simulink model "Compensator"  (Simulink 6.1)
settings: Solver=ode45  StartTime=0.0  StopTime=10.0  RelTol=1e-3
libraries: dspmtrx3 x2
settings Model: LastModifiedBy=fhuang
settings DebuggingCC: SolverPrmCheckMsg=warning

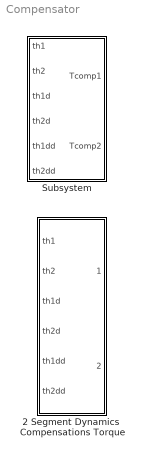
== system Compensator ==
  2 Segment Dynamics  Compensations Torque : Subsystem
  Subsystem : Subsystem

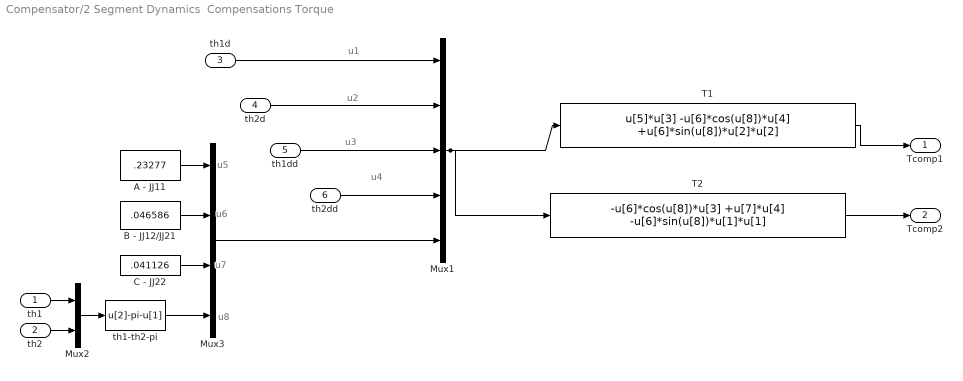
== system Compensator/2 Segment Dynamics  Compensations Torque ==
  note: u1
  note: u2
  note: u3
  note: u4
  note: u5
  note: u6
  note: u7
  note: u8
  th1 : Inport  Port=1  LatchInput=off
  th2 : Inport  Port=2  LatchInput=off
  th1d : Inport  Port=3  LatchInput=off
  th2d : Inport  Port=4  LatchInput=off
  th1dd : Inport  Port=5  LatchInput=off
  th2dd : Inport  Port=6  LatchInput=off
  A - JJ11 : Constant  Value=.23277
  B - JJ12/JJ21 : Constant  Value=.046586
  C - JJ22 : Constant  Value=.041126
  Mux1 : Mux  Inputs=5
  Mux2 : Mux  Inputs=2
  Mux3 : Mux
  T1 : Fcn  Expr="u[5]*u[3]   -u[6]*cos(u[8])*u[4]   +u[6]*sin(u[8])*u[2]*u[2]"
  T2 : Fcn  Expr="-u[6]*cos(u[8])*u[3]    +u[7]*u[4]    -u[6]*sin(u[8])*u[1]*u[1]"
  th1-th2-pi : Fcn  Expr=u[2]-pi-u[1]
  Tcomp1 : Outport
  Tcomp2 : Outport  Port=2
  wires:
  T1/1 -> Tcomp1/1
  Mux1/1 -> T1/1, T2/1
  Mux3/1 -> Mux1/5
  A - JJ11/1 -> Mux3/1
  B - JJ12/JJ21/1 -> Mux3/2
  C - JJ22/1 -> Mux3/3
  th1-th2-pi/1 -> Mux3/4
  th1d/1 -> Mux1/1
  th2d/1 -> Mux1/2
  th1dd/1 -> Mux1/3
  th2dd/1 -> Mux1/4
  th2/1 -> Mux2/2
  th1/1 -> Mux2/1
  Mux2/1 -> th1-th2-pi/1
  T2/1 -> Tcomp2/1

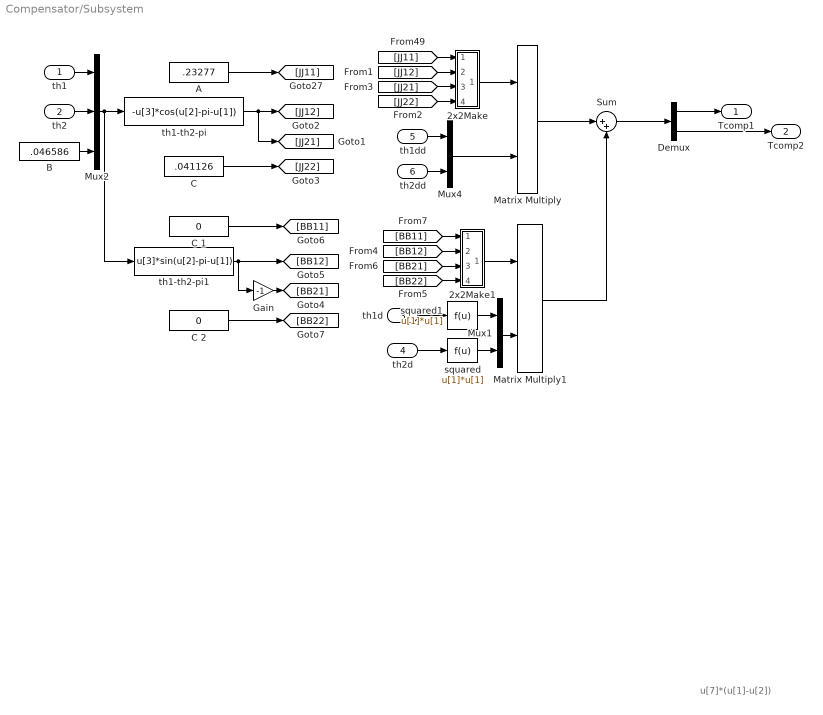
== system Compensator/Subsystem ==
  note: u[7]*(u[1]-u[2])
  th1 : Inport  Port=1  LatchInput=off
  th2 : Inport  Port=2  LatchInput=off
  th1d : Inport  Port=3  LatchInput=off
  th2d : Inport  Port=4  LatchInput=off
  th1dd : Inport  Port=5  LatchInput=off
  th2dd : Inport  Port=6  LatchInput=off
  2x2Make : Subsystem
  2x2Make1 : Subsystem
  A : Constant  Value=.23277
  B : Constant  Value=.046586
  "C " : Constant  Value=.041126
  C 1 : Constant  Value=0
  C 2 : Constant  Value=0
  Demux : Demux  Outputs=2
  Gain : Gain  Gain=-1
  Matrix Multiply : dspmtrx3/Matrix Multiply  numInputPorts=2  OptimizationLevel=None
  Matrix Multiply1 : dspmtrx3/Matrix Multiply  numInputPorts=2  OptimizationLevel=None
  Mux1 : Mux  Inputs=2
  Mux2 : Mux  Inputs=3
  Mux4 : Mux  Inputs=2
  Sum : Sum  Inputs=|++
  squared : Fcn  Expr=u[1]*u[1]
  squared1 : Fcn  Expr=u[1]*u[1]
  th1-th2-pi : Fcn  Expr=-u[3]*cos(u[2]-pi-u[1])
  th1-th2-pi1 : Fcn  Expr=u[3]*sin(u[2]-pi-u[1])
  Tcomp1 : Outport
  Tcomp2 : Outport  Port=2
  wires:
  th2d/1 -> squared/1
  th1dd/1 -> Mux4/1
  th2dd/1 -> Mux4/2
  th2/1 -> Mux2/2
  th1/1 -> Mux2/1
  Mux2/1 -> th1-th2-pi/1, th1-th2-pi1/1
  A/1 -> [JJ11]
  B/1 -> Mux2/3
  th1-th2-pi/1 -> [JJ12], [JJ21]
  "C "/1 -> [JJ22]
  [JJ11] -> 2x2Make/1(In1)
  [JJ12] -> 2x2Make/2(In2)
  [JJ21] -> 2x2Make/3(In3)
  [JJ22] -> 2x2Make/4(In4)
  2x2Make/1(Out1) -> Matrix Multiply/1
  Mux4/1 -> Matrix Multiply/2
  [BB11] -> 2x2Make1/1(In1)
  [BB12] -> 2x2Make1/2(In2)
  [BB21] -> 2x2Make1/3(In3)
  [BB22] -> 2x2Make1/4(In4)
  th1d/1 -> squared1/1
  2x2Make1/1(Out1) -> Matrix Multiply1/1
  Mux1/1 -> Matrix Multiply1/2
  C 2/1 -> [BB22]
  th1-th2-pi1/1 -> [BB12], Gain/1
  C 1/1 -> [BB11]
  Gain/1 -> [BB21]
  Matrix Multiply/1 -> Sum/1
  Matrix Multiply1/1 -> Sum/2
  squared/1 -> Mux1/2
  squared1/1 -> Mux1/1
  Sum/1 -> Demux/1
  Demux/1 -> Tcomp1/1
  Demux/2 -> Tcomp2/1

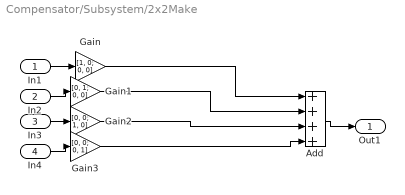
== system Compensator/Subsystem/2x2Make ==
  In1 : Inport  Port=1  LatchInput=off
  In2 : Inport  Port=2  LatchInput=off
  In3 : Inport  Port=3  LatchInput=off
  In4 : Inport  Port=4  LatchInput=off
  Add : Sum  Inputs=++++  OutScaling=2^-10
  Gain : Gain  Gain=[1, 0; 0, 0]
  Gain1 : Gain  Gain=[0, 1; 0, 0]
  Gain2 : Gain  Gain=[0, 0; 1, 0]
  Gain3 : Gain  Gain=[0, 0; 0, 1]
  Out1 : Outport
  wires:
  Add/1 -> Out1/1
  Gain/1 -> Add/1
  Gain1/1 -> Add/2
  Gain2/1 -> Add/3
  Gain3/1 -> Add/4
  In1/1 -> Gain/1
  In2/1 -> Gain1/1
  In3/1 -> Gain2/1
  In4/1 -> Gain3/1

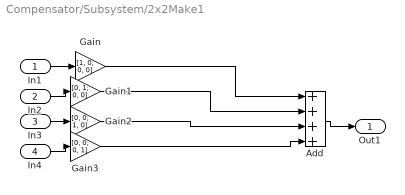
== system Compensator/Subsystem/2x2Make1 ==
  In1 : Inport  Port=1  LatchInput=off
  In2 : Inport  Port=2  LatchInput=off
  In3 : Inport  Port=3  LatchInput=off
  In4 : Inport  Port=4  LatchInput=off
  Add : Sum  Inputs=++++  OutScaling=2^-10
  Gain : Gain  Gain=[1, 0; 0, 0]
  Gain1 : Gain  Gain=[0, 1; 0, 0]
  Gain2 : Gain  Gain=[0, 0; 1, 0]
  Gain3 : Gain  Gain=[0, 0; 0, 1]
  Out1 : Outport
  wires:
  In4/1 -> Gain3/1
  In3/1 -> Gain2/1
  In2/1 -> Gain1/1
  In1/1 -> Gain/1
  Gain3/1 -> Add/4
  Gain2/1 -> Add/3
  Gain1/1 -> Add/2
  Gain/1 -> Add/1
  Add/1 -> Out1/1
